simulink model "ValidateROMBatteryModel"  (R2024b)
settings: Solver=VariableStepAuto  StartTime=0.0  StopTime=1068  FixedStep=0.1  RelTol=1e-3
PreLoadFcn:
  | % Load parameters
  | load ModelData.mat;
  | 
  | % Load an independent current profile
  | load Artemis150mphCurrent_TS.mat;
  | 
  | % Load trained NLARX model
  | load NLARXModel.mat;
values from neighbouring files (symbols this model uses):
  Np = 4    [ModuleExample_ref.m]
undefined symbols (not defined in the file or in its folder): AH, SOCs, Ts
libraries: fl_lib x6, nesl_utility x2, slident x1, batt_lib x1, moduleExample_lib x1, SimscapeFluids_lib x1
settings Model: Creator=kmahadev  LastModifiedBy=kmahadev
settings OptimizationCC: DefaultParameterBehavior=Inlined  EnhancedBackFolding=on  PassReuseOutputArgsAs=Individual arguments  ZeroExternalMemoryAtStartup=off  ZeroInternalMemoryAtStartup=off  OptimizeBlockOrder=speed  DifferentSizesBufferReuse=on  OptimizationCustomize=off  EfficientTunableParamExpr=on
settings DebuggingCC: ParameterTunabilityLossMsg=error
settings SFSimCC: MATLABDynamicMemAlloc=off
settings RTWCC: Description=Embedded Coder  SystemTargetFile=ert.tlc  TemplateMakefile=ert_default_tmf  TargetLang=C++
settings CodeAppCC: ForceParamTrailComments=on  IgnoreCustomStorageClasses=off  OperatorAnnotations=on  SimulinkDataObjDesc=on  SFDataObjDesc=on  InsertBlockDesc=on
settings ERTTargetCC: TargetLangStandard=C++11 (ISO)  GenerateSampleERTMain=on  CodeInterfacePackaging=C++ class  RootIOFormat=Structure reference  ERTCustomFileTemplate=example_file_process.tlc  DynamicArrayContainerType=coder::array

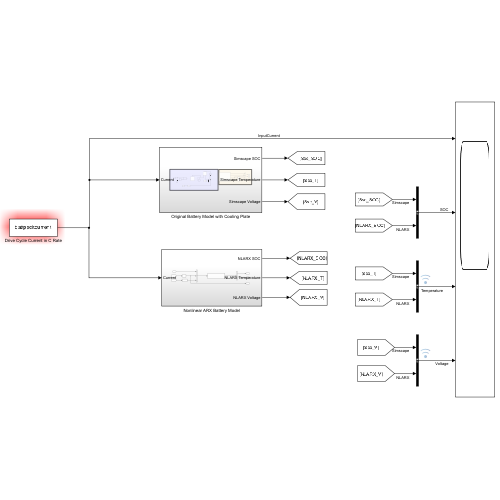
[thumbnail: Simulink's stored preview of the top-level diagram]
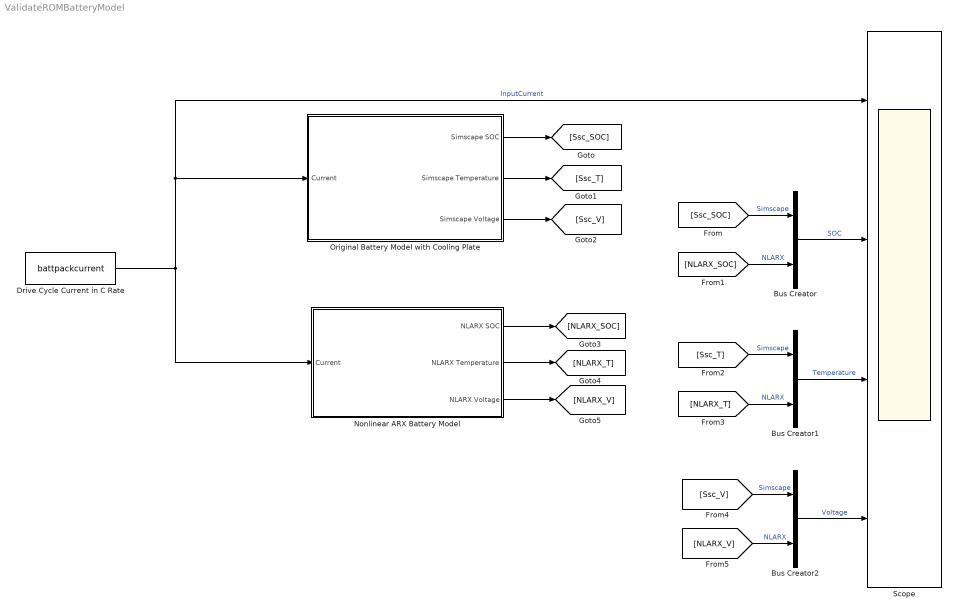
== system ValidateROMBatteryModel ==
  Bus Creator : BusCreator  Inputs=2
  Bus Creator1 : BusCreator  Inputs=2
  Bus Creator2 : BusCreator  Inputs=2
  Drive Cycle Current in C Rate : FromWorkspace  VariableName=battpackcurrent
  Nonlinear ARX Battery Model : Subsystem
  Original Battery Model with Cooling Plate : Subsystem
  Scope : Scope  NumInputPorts=4
  wires:
  Bus Creator2/1 -> Scope/4  "Voltage"
  [Ssc_T] -> Bus Creator1/1  "Simscape"
  Nonlinear ARX Battery Model/1(NLARX SOC) -> [NLARX_SOC]
  Nonlinear ARX Battery Model/2(NLARX Temperature) -> [NLARX_T]
  Original Battery Model with Cooling Plate/1(Simscape SOC) -> [Ssc_SOC]
  Drive Cycle Current in C Rate/1 -> Nonlinear ARX Battery Model/1(Current), Original Battery Model with Cooling Plate/1(Current), Scope/1  "InputCurrent"
  [Ssc_V] -> Bus Creator2/1  "Simscape"
  Original Battery Model with Cooling Plate/3(Simscape Voltage) -> [Ssc_V]
  Bus Creator1/1 -> Scope/3  "Temperature"
  Nonlinear ARX Battery Model/3(NLARX Voltage) -> [NLARX_V]
  [Ssc_SOC] -> Bus Creator/1  "Simscape"
  [NLARX_T] -> Bus Creator1/2  "NLARX"
  Bus Creator/1 -> Scope/2  "SOC"
  Original Battery Model with Cooling Plate/2(Simscape Temperature) -> [Ssc_T]
  [NLARX_SOC] -> Bus Creator/2  "NLARX"
  [NLARX_V] -> Bus Creator2/2  "NLARX"

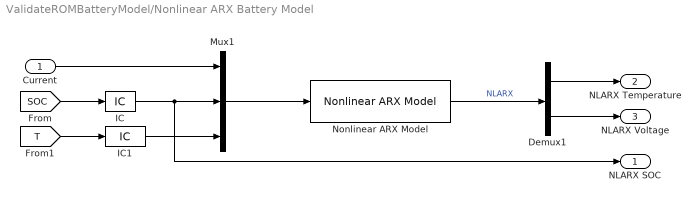
== system ValidateROMBatteryModel/Nonlinear ARX Battery Model ==
  Current : Inport
  Demux1 : Demux  Outputs=2
  IC : InitialCondition  Value=SOCs
  IC1 : InitialCondition  Value=Ts
  Mux1 : Mux  Inputs=3
  Nonlinear ARX Model : slident/Models/Nonlinear ARX Model  sys=NLARX_trainingOutput.NonlinearModel  ICspec=Input and output values  X0="[0.5 0.5 SOCs SOCs SOCs Ts Ts  Ts Ts]"  U0=[0.5 SOCs Ts]  Y0=[Ts 36.96]
  NLARX SOC : Outport
  NLARX Temperature : Outport  Port=2
  NLARX Voltage : Outport  Port=3
  wires:
  IC/1 -> NLARX SOC/1, Mux1/2
  [T] -> IC1/1
  [SOC] -> IC/1
  IC1/1 -> Mux1/3
  Demux1/1 -> NLARX Temperature/1
  Mux1/1 -> Nonlinear ARX Model/1
  Nonlinear ARX Model/1 -> Demux1/1  "NLARX"
  Current/1 -> Mux1/1
  Demux1/2 -> NLARX Voltage/1

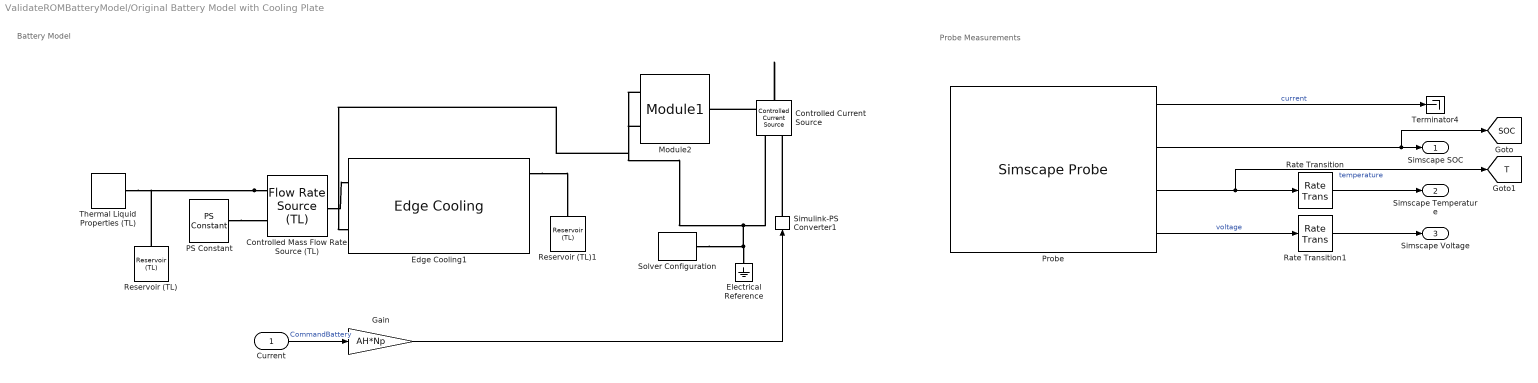
== system ValidateROMBatteryModel/Original Battery Model with Cooling Plate ==
  note: Probe Measurements
  note: Battery Model
  Current : Inport
  Controlled Current Source : fl_lib/Electrical/Electrical Sources/Controlled Current Source
  Controlled Mass Flow Rate Source (TL) : fl_lib/Thermal Liquid/Sources/Flow Rate Source (TL)  source_type=foundation.enum.constant_controlled.controlled  flow_type=foundation.enum.mass_volumetric_flow.mass  mass_flow=0 kg/s  volumetric_flow=0 m^3/s  power_spec=foundation.enum.power_spec.isentropic  area=0.01 m^2
  Edge Cooling1 : batt_lib/Thermal/Edge Cooling  plateConnectivity=simscape.battery.enum.thermal.coolingPlateConnectivity.singleSided  numBattThermalNodes1=module.ThermalNodes.Bottom.NumNodes  dimensionThermalNodes1=module.ThermalNodes.Bottom.Dimensions  locationThermalNodes1=module.ThermalNodes.Bottom.Locations  numBattThermalNodes2=1  dimensionThermalNodes2=ones(1, 2)  locationThermalNodes2=ones(1, 2)  plateDimX=2  plateDimY=5  plateTh=2e-3 m  plateThCond=20 W/(K*m)  plateDen=2500 kg/m^3  plateCp=447 J/(K*kg)  plateTemp_ini=278 K  Re_lam=2000  Re_tur=4000  Nu_lam=3.66  length_add=1e-3 m  shape_factor=64  selectEdgeOrientation=simscape.battery.enum.thermal.coolingEdgeDirection.alongY0  channelDia=5e-3 m  channelArea=2e-5 m^2  roughnessPipe=1.5e-05 m
      settings: InternalSimscapePortConfiguration="{\"Bottom\":[],\"Left\":[{\"id\":\"fluid_in\",\"label\":\"fluid_in\",\"type\":\"foundation.thermal_liquid.thermal_liquid\"}],\"Right\":[{\"id\":\"fluid_out\",\"label\":\"fluid_out\",\"type\":\"foundation.thermal_liquid.thermal_liquid\"},{\"id\":\"plotPlateT\",\"label\":\"Tp\",\"type\":\"output\"},{\"id\":\"tempSensor\",\"label\":\"dT\",\"type\":\"output\"},{\"id\":\"presSensor\",\"label\":\"dP\",\"type\":\"output\"}],\"Top\":[{\"id\":\"Side1\",\"label\":\"Surf1\",\"type\":\"foundation.thermal.thermal\"}]}"
  Electrical Reference : fl_lib/Electrical/Electrical Elements/Electrical Reference
  Gain : Gain  Gain=AH*Np
  Module2 : moduleExample_lib/Module1  SOC_vec=[0, .1, .25, .5, .75, .9, 1]  T_vec=[278, 293, 313] K  V0_mat=[3.49, 3.5, 3.51; 3.55, 3.57, 3.56; 3.62, 3.63, 3.64; 3.71, 3.71, 3.72; 3.91, 3.93, 3.94; 4.07, 4.08, 4.08; 4.19, 4.19, 4.19] V  V_range=[0, inf] V  R0_mat=[.0117, .0085, .009; .011, .0085, .009; .0114, .0087, .0092; .0107, .0082, .0088; .0107, .0083, .0091; .0113, .0085, .0089; .0116, .0085, .0089] Ohm  AH=27 A*hr  extrapolation_option=simscape.enum.extrapolation.nearest  R1_mat=[.0109, .0029, .0013; .0069, .0024, .0012; .0047, .0026, .0013; .0034, .0016, .001; .0033, .0023, .0014; .0033, .0018, .0011; .0028, .0017, .0011] Ohm  tau1_mat=[20, 36, 39; 31, 45, 39; 109, 105, 61; 36, 29, 26; 59, 77, 67; 40, 33, 29; 25, 39, 33] s  thermal_mass=100 J/K  CoolantResistance=1.2 K/W  P=4  S=10  iCellModel_specify=off  iCellModel_priority=None  iCellModel=0 A  iCellModel_nominal_specify=off  iCellModel_nominal_unit=A  iCellModel_nominal_value=1  vCellModel_specify=off  vCellModel_priority=None  vCellModel=0 V  vCellModel_nominal_specify=off  vCellModel_nominal_unit=V  vCellModel_nominal_value=1  socCellModel_specify=on  socCellModel_priority=High  socCellModel=SOCs  socCellModel_nominal_specify=off  socCellModel_nominal_unit=1  socCellModel_nominal_value=1  numCyclesCellModel_specify=off  numCyclesCellModel_priority=High  numCyclesCellModel=0  numCyclesCellModel_nominal_specify=off  numCyclesCellModel_nominal_unit=1  numCyclesCellModel_nominal_value=1  temperatureCellModel_specify=on  temperatureCellModel_priority=High  temperatureCellModel=Ts K  temperatureCellModel_nominal_specify=off  temperatureCellModel_nominal_unit=K  temperatureCellModel_nominal_value=1  vParallelAssembly_specify=off  vParallelAssembly_priority=None  vParallelAssembly=repmat(0, 10, 1) V  vParallelAssembly_nominal_specify=off  vParallelAssembly_nominal_unit=V  vParallelAssembly_nominal_value=1  socParallelAssembly_specify=off  socParallelAssembly_priority=None  socParallelAssembly=repmat(1, 10, 1)  socParallelAssembly_nominal_specify=off  socParallelAssembly_nominal_unit=1  socParallelAssembly_nominal_value=1
      settings: InternalSimscapePortConfiguration="{\"Bottom\":[{\"id\":\"n\",\"label\":\"-\",\"type\":\"foundation.electrical.electrical\"},{\"id\":\"BottomExtClnt\",\"label\":\"CPB\",\"type\":\"foundation.thermal.thermal\"}],\"Left\":[],\"Right\":[],\"Top\":[{\"id\":\"p\",\"label\":\"+\",\"type\":\"foundation.electrical.electrical\"}]}"
  PS Constant : fl_lib/Physical Signals/Sources/PS Constant  constant=0.2 kg/s
  Probe : SimscapeProbe  BoundBlock=68  Variables={iCellModel, socCellModel, temperatureCellModel, vCellModel}
  Rate Transition : RateTransition  InitialCondition=Ts  OutPortSampleTime=0.1
  Rate Transition1 : RateTransition  InitialCondition=38  OutPortSampleTime=0.1
  Reservoir (TL) : fl_lib/Thermal Liquid/Elements/Reservoir (TL)  pressure_spec=foundation.enum.pressure_spec.atmospheric  reservoir_pressure=0.101325 MPa  reservoir_temperature=278 K  area=0.01 m^2
  Reservoir (TL)1 : fl_lib/Thermal Liquid/Elements/Reservoir (TL)  pressure_spec=foundation.enum.pressure_spec.atmospheric  reservoir_pressure=0.101325 MPa  reservoir_temperature=278 K  area=0.01 m^2
  Simulink-PS Converter1 : nesl_utility/Simulink-PS Converter  PhysicalDomain=network_engine_domain  SubClassName=ps_input  LeftPortType=input  RightPortType=output  PseudoPeriodic=off  Frequencies=[]  NoiseDistribution=none  NoiseParameters=[]  Unit=1  AffineConversion=off  FilteringAndDerivatives=provide  SimscapeFilterOrder=1  InputFilterTimeConstant=0.001  UdotUserProvided=0
  Solver Configuration : nesl_utility/Solver Configuration  PhysicalDomain=network_engine_domain  SubClassName=solver  LeftPortType=input  RightPortType=generic  Tones=[]  Harmonics=[]  SimulateNoise=off  Profile=off  UseLocalSampling=off  EnableSwitchedLinearOptims=on  FrequencyDomain=off  UseCCode=off  RelTol=0.001  AbsTol=0.001  MinStep=1e-09  ToWorkspace=off  RevertToSquareIcSolve=off  NumHomotopyIterations=100  PhasorMode=off  PhasorModeNumHarmonics=1  ConsistencySolver=NEWTON_XTOL_AFTER_FTOL  IndexReductionMethod=DerivativeReplacement  DoDC=off  ResidualTolerance=1e-09  ConsistencyTolSource=GLOBAL  ConsistencyAbsTol=0.001  ConsistencyRelTol=0.001  ConsistencyTolFactor=0.001  UseLocalSolver=off  LocalSolverChoice=NE_BACKWARD_EULER_ADVANCER  ResolveIndetEquations=on  FunctionEvalNumThread=1  LocalSolverSampleTime=0.001  DoFixedCost=off  MaxNonlinIter=3  MaxModeIter=2  ComputeImpulses=off  ImpulseIterations=2  LinearAlgebra=auto  LinearAlgebraNumThread=0  EquationFormulation=NE_TIME_EF  DelaysMemoryBudget=1024  AutomaticFiltering=on  FilteringTimeConstant=0.001  PartitionStorageMethod=AS_NEEDED  PartitionMemoryBudget=1024  PartitionMethod=ROBUST  MultibodyUseLocalSolver=off  MultibodyLocalSolverChoice=ODE1  MultibodyLocalSolverSampleTime=0.001
  Terminator4 : Terminator
  Thermal Liquid Properties (TL) : SimscapeFluids_lib/Thermal Liquid/Utilities/Thermal Liquid Properties (TL)  fluid_list=fluids.thermal_liquid.utilities.enum.thermal_liquid_fluid_list.water  concentration_param_EG=fluids.thermal_liquid.utilities.enum.thermal_liquid_concentration.volume_fraction  concentration_param_PG=fluids.thermal_liquid.utilities.enum.thermal_liquid_concentration.volume_fraction  c_mass_SW=3.5e-3  c_mass_EG=0.1  c_mass_PG=0.1  c_mass_GL=0.1  c_vol_EG=0.1  c_vol_PG=0.1  beta_const_EG=2.1791 GPa  beta_const_PG=2.1791 GPa  beta_const_GL=2.1791 GPa  p_min_EG=0.01 MPa  p_min_PG=0.01 MPa  p_min_GL=0.01 MPa  p_max_EG=50 MPa  p_max_PG=50 MPa  p_max_GL=50 MPa  p_atm=0.101325 MPa  properties_range_check=simscape.enum.assert.action.error
  Simscape SOC : Outport
  Simscape Temperature : Outport  Port=2
  Simscape Voltage : Outport  Port=3
  tag scope: SOC=global, T=global
  wires:
  Probe/4 -> Rate Transition1/1  "voltage"
  Probe/3 -> [T], Rate Transition/1  "temperature"
  Rate Transition/1 -> Simscape Temperature/1
  Rate Transition1/1 -> Simscape Voltage/1
  Probe/2 -> [SOC], Simscape SOC/1
  Probe/1 -> Terminator4/1  "current"
  Gain/1 -> Simulink-PS Converter1/1
  Current/1 -> Gain/1  "CommandBattery"
  connections:
  Solver Configuration/RConn1 -- Module2/RConn1 -- Controlled Current Source/RConn2 -- Electrical Reference/LConn1
  Controlled Mass Flow Rate Source (TL)/LConn1 -- Reservoir (TL)/LConn1 -- Thermal Liquid Properties (TL)/RConn1
  Module2/RConn2 -- Edge Cooling1/LConn2
  Simulink-PS Converter1/RConn1 -- Controlled Current Source/RConn1
  Controlled Current Source/LConn1 -- Module2/LConn1
  Controlled Mass Flow Rate Source (TL)/RConn1 -- Edge Cooling1/LConn1
  Edge Cooling1/RConn1 -- Reservoir (TL)1/LConn1
  PS Constant/RConn1 -- Controlled Mass Flow Rate Source (TL)/LConn2
